simulink model "SVPWM_Simulation"  (R2018a)
settings: Solver=ode5  StartTime=0.0  StopTime=10  FixedStep=50e-6  MaxStep=1e-6  RelTol=1e-3  EnableMultiTasking=on
PostLoadFcn:
  | , if any(exist('dsrtsu_mdlpostloadfcn', 'file') == [2, 3, 6]), try dsrtsu_mdlpostloadfcn('Execute', bdroot); catch fprintf('Error in PostLoadFcn (dsrtsu_mdlpostloadfcn) for model "%s":\n %s\n', bdroot, lasterr); end, end,
InitFcn:
  | clear;
  | clc;
libraries: powerlib x8, simulink x1
settings Model: DSRTSU_INTERNAL_RTI_VER=510  DSRTSU_INTERNAL_RTI_TYPE=rti1104  RTICANMMDATA=struct('GeneralSetupData',struct('modelroot','C:\Users\elec\Desktop\SVPWM_1','generalsettings',struct('filesettings',struct('destfolder',struct('Name','RTICANMM_FILES','Check',1),'buildfolder',struct('Name','.','Check',1),'AbsDestfolder',struct('Name','C:\Users\elec\Desktop\SVPWM_1\RTICANMM_FILES'),'AbsBuildfolder',struct('Name','C:\Users\elec\Desktop\SVPWM_1'))),'options',struct('addpaths',1,'rmpaths',1,'addtrcexclusion',logical(1),'cannavigator',struct('checkmonitoring',0),'show_usrtrc',0,'use_usrtrc',0),'advanced',struct('options',[1 1 1 1 1 1 1 1 1 1 1 1 1 1 1 1 1 1 1 1 1 1 1 1 1 1 1 1 1 1 1 1 1 1 1 1 1 1 1 1 1 1 1 1 1 1 1 1 1 1 1 1 1 1 1 1 1 1 1 1 1 1 1 1 1 1 1 1 1 1 1 1 1 1 1 1 1 1 1 1 1 1 1 1 1 1 1 1 1 1 1 1 1 1 1 1 1 1 1 1]),'MPSetup',{{}},'modelname','shashank','block','shashank'))  DSRTSU_INTERNAL_RTIFLEXRAYCONFIG=110  DSRTSU_INTERNAL_RTIFPGA=110  Creator=HP  LastModifiedBy=asus
settings DataIOCC: LimitDataPoints=on  SaveFormat=Array
settings OptimizationCC: BlockReduction=off  ExpressionDepthLimit=2147483647
settings DebuggingCC: UnderspecifiedInitializationDetection=Classic  MergeDetectMultiDrivingBlocksExec=none  SolverPrmCheckMsg=warning  FcnCallInpInsideContextMsg=warning  StateNameClashWarn=warning  SFUnexpectedBacktrackingDiag=warning  SFNoUnconditionalDefaultTransitionDiag=warning  SFExecutionAtInitializationDiag=none
settings HardwareCC: ProdBitPerPointer=32  ProdBitPerSizeT=32  ProdBitPerPtrDiffT=32  ProdLargestAtomicInteger=Integer  ProdEndianess=BigEndian  ProdWordSize=32  ProdHWDeviceType=Custom Processor->Custom  TargetIntDivRoundTo=Zero  TargetEndianess=BigEndian  TargetHWDeviceType=Custom Processor->Custom
settings ModelReferenceCC: PropagateSignalLabelsOutOfModel=off
settings SFSimCC: MATLABDynamicMemAlloc=off
settings RTWCC: SystemTargetFile=rti1104.tlc  MakeCommand=make_rti  TemplateMakefile=rti1104.tmf  Description=dSPACE DS1104 Hardware Platform
settings CodeAppCC: StateflowObjectComments=on
settings STFCustomTargetCC: ParMdlRefBuildCompliant=on  GRTInterface=off  SystemTargetFile=rti1104.tlc
settings GRTTargetCC: TargetLangStandard=C89/C90 (ANSI)  CompOptLevelCompliant=off  ConcurrentExecutionCompliant=off  CombineOutputUpdateFcns=off  MatFileLogging=off  CPPClassGenCompliant=off  UseToolchainInfoCompliant=off
settings ConfigComp: CovMetricSettings=dw  CovHtmlReporting=on  CovSaveCumulativeToWorkspaceVar=on  CovSaveSingleToWorkspaceVar=on  CovExternalEMLEnable=off
settings SimscapeCC: SimscapeNormalizeSystem=off

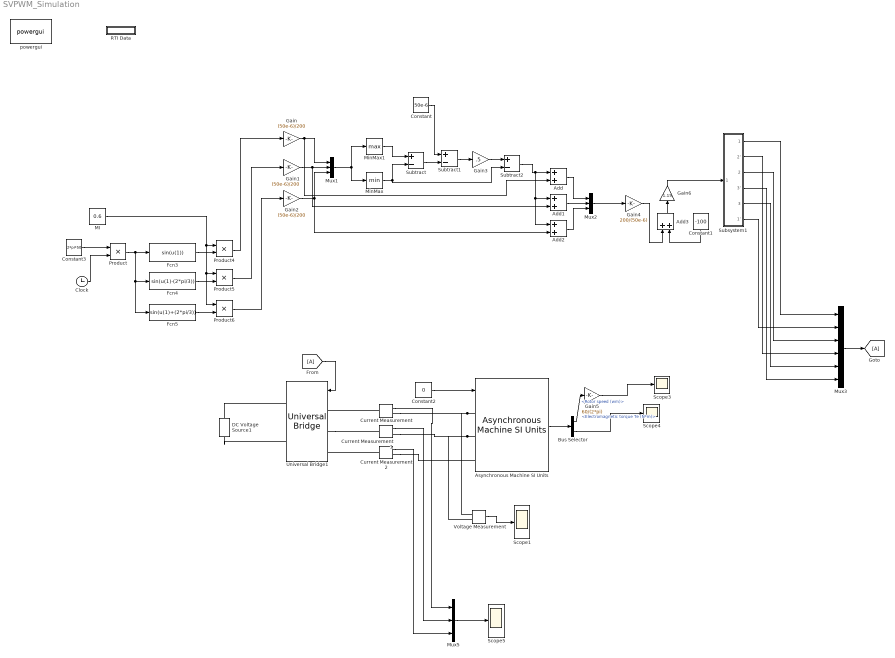
== system SVPWM_Simulation ==
  Add{,1..3} (4 alike) : Sum
  Asynchronous Machine SI Units : powerlib/Machines/Asynchronous Machine SI Units  RotorType=Squirrel-cage  PresetModel=No  MechanicalLoad=Torque Tm  ShowDetailedParameters=on  ReferenceFrame=Rotor  Units=SI  MeasurementBus=off  NominalParameters=[1300 415 50]  Stator=[14.15 0.0435]  Rotor=[4.36 0.0435]  Cage1=[ 0.022 0.226/377]  Cage2=[ 0.022 0.226/377]  Lm=0.59  Mechanical=[0.0131 0.002985 2]  PolePairs=2  InitialConditions=[1 0 0 0 0 0 0 0]  SimulateSaturation=off  Saturation=[14.03593122, 27.81365428, 53.79336849, 72.68890987, 97.98006896, 148.6815601, 215.7428561, 302.9841135, 428.7778367 ; 230, 322, 414, 460, 506, 552, 598, 644, 690]  LoadFlowParameters=1492000  TsPowergui=0  TsBlock=-1  IterativeModel=Trapezoidal non iterative  IterativeDiscreteModel=Trapezoidal non iterative  Pmec=0
  Bus Selector : BusSelector  OutputSignals=Mechanical.Rotor speed (wm),Mechanical.Electromagnetic torque Te (N*m)
  Clock : Clock
  Constant : Constant  Value=50e-6
  Constant1 : Constant  Value=-100
  Constant2 : Constant  Value=0
  Constant3 : Constant  Value=2*pi*50
  Current Measurement : powerlib/Measurements/Current Measurement  PhasorSimulation=off  OutputType=Complex  PSBequivalent=0
  Current Measurement1 : powerlib/Measurements/Current Measurement  PhasorSimulation=off  OutputType=Complex  PSBequivalent=0
  Current Measurement2 : powerlib/Measurements/Current Measurement  PhasorSimulation=off  OutputType=Complex  PSBequivalent=0
  DC Voltage Source1 : powerlib/Electrical Sources/DC Voltage Source  Amplitude=200  Measurements=None
  Fcn3 : Fcn  Expr=sin(u(1))
  Fcn4 : Fcn  Expr=sin(u(1)-(2*pi/3))
  Fcn5 : Fcn  Expr=sin(u(1)+(2*pi/3))
  Gain : Gain  Gain=(50e-6)/200
  Gain1 : Gain  Gain=(50e-6)/200
  Gain2 : Gain  Gain=(50e-6)/200
  Gain3 : Gain  Gain=.5
  Gain4 : Gain  Gain=200/(50e-6)
  Gain5 : Gain  Gain=60/(2*pi)
  Gain6 : Gain  Gain=1.15
  MI : Constant  Value=0.6
  MinMax : MinMax
  MinMax1 : MinMax  Function=max
  Mux1 : Mux  Inputs=3
  Mux2 : Mux  Inputs=3
  Mux3 : Mux  Inputs=6
  Mux5 : Mux  Inputs=3
  Product : Product
  Product4 : Product  RndMeth=Zero
  Product5 : Product  RndMeth=Zero
  Product6 : Product  RndMeth=Zero
  RTI Data : Subsystem  Tag=struct('RTIDataServer',struct('RTIDataServerVs','2','RTIModelDescription','struct(''main'',''shashank_load'',''sub'',''shashank_load'',''isMp'',0)'))  LoadFcn="if exist('rtidc'), try,  rtidc('DataHostBlockClbLoad', gcbh); catch, disp(['Warning: ''LoadFcn'' for RTI Data block failed: ' lasterr]); end, end,"  mask(RTI_DATA_HOST){}
      mask help:
      | RTI Data Block.
      | This block is used by RTI to store internal model-dependent data.
      | Please keep this block on the root level of the model. Deleting this block will result in data loss.
      |
      | NEVER DELETE OR COPY THIS BLOCK!
      settings: CopyFcn="if exist('rtidc'), try,  rtidc('DataHostBlockClbCopy', gcbh); catch, disp(['Warning: ''CopyFcn'' for RTI Data block failed: ' lasterr]); end, end,"  DeleteFcn="if exist('rtidc'), try,  rtidc('DataHostBlockClbDelete', gcbh); catch, disp(['Warning: ''DeleteFcn'' for RTI Data block failed: ' lasterr]); end, end,"  ModelCloseFcn="if exist('rtidc'), try,  rtidc('DataHostBlockClbModelClose', gcbh); catch, disp(['Warning: ''ModelCloseFcn'' for RTI Data block failed: ' lasterr]); end, end,"  PreSaveFcn="if exist('rtidc'), try,  rtidc('DataHostBlockClbPreSave', gcbh); catch, disp(['Warning: ''PreSaveFcn'' for RTI Data block failed: ' lasterr]); end, end,"  PostSaveFcn="if exist('rtidc'), try,  rtidc('DataHostBlockClbPostSave', gcbh); catch, disp(['Warning: ''PostSaveFcn'' for RTI Data block failed: ' lasterr]); end, end,"  NameChangeFcn="if exist('rtidc'), try,  rtidc('DataHostBlockClbNameChange', gcbh); catch, disp(['Warning: ''NameChangeFcn'' for RTI Data block failed: ' lasterr]); end, end,"
      mask Help:
      | RTI Data Block.
      | This block is used by RTI to store internal model-dependent data.
      | Please keep this block on the root level of the model. Deleting this block will result in data loss.
      | 
      | NEVER DELETE OR COPY THIS BLOCK!
      mask Display:
      | text(0.5, 0.5, 'RTI Data', 'HorizontalAlignment', 'center');
      | plot([1 0]);
  Scope{1,3..5} (4 alike) : Scope
  Subsystem1 : Subsystem
  Subtract : Sum  Inputs=+-
  Subtract1 : Sum  Inputs=+-
  Subtract2 : Sum  Inputs=+-
  Universal Bridge1 : powerlib/Power Electronics/Universal Bridge  Arms=3  SnubberResistance=1e5  SnubberCapacitance=inf  Device=IGBT / Diodes  Ron=1e-3  Lon=0  ForwardVoltages="[  0  0  ]"  ForwardVoltage=0  GTOparameters=[ 10e-6 , 20e-6 ]  IGBTparameters=[ 1e-6 , 2e-6 ]  Measurements=None  Measurements_2=None  converterType=Rectifier
  Voltage Measurement : powerlib/Measurements/Voltage Measurement  PhasorSimulation=off  OutputType=Complex  PSBequivalent=0
  powergui : powerlib/powergui  Priority=1  SimulationMode=Discrete  SampleTime=50e-6  frequency=60  Iterations=50  frequencyindice=0  Pbase=100e6  ErrMax=1e-4  UnitsV=kV  UnitsW=MW  buscounter=0  FunctionMessages=off  echomessages=off  EnableUseOfTLC=off  CurrentSourceSwitches=off  DisableSnubberDevices=off  DisableRonSwitches=off  DisableVfSwitches=off  DisplayEquations=off  SolverType=Tustin  Interpol=off  ExternalGateDelay=off  methode=off  Ts=0  x0status=blocks  SPID=off  SwTol=0  HookPort=off  RestoreLinks=warning  ResistiveCurrentMeasurement=off  Frange=[0:2:500]  Ylog=off  Xlog=on  ShowGrid=off  save=off  variable=ZData  structure=a5  ZoomFFT=off  StartTime=.2  cycles=3  DisplayStyle=2  fundamental=50  FreqAxis=on  MaxFrequency=1000  frequencyindicesteady=1  RmsSteady=1  display=off
  wires:
  Subtract1/1 -> Gain3/1
  Constant3/1 -> Product/1
  Mux1/1 -> MinMax1/1, MinMax/1
  MI/1 -> Product6/1, Product5/1, Product4/1
  Fcn5/1 -> Product6/2
  Product/1 -> Fcn5/1, Fcn4/1, Fcn3/1
  MinMax/1 -> Subtract/2, Subtract2/2
  Fcn4/1 -> Product5/2
  Product4/1 -> Gain/1
  Gain1/1 -> Mux1/2, Add1/2
  Constant1/1 -> Add3/2
  Clock/1 -> Product/2
  Gain2/1 -> Mux1/3, Add2/2
  Mux2/1 -> Gain4/1
  Subtract2/1 -> Add/1, Add1/1, Add2/1
  MinMax1/1 -> Subtract/1
  Gain6/1 -> Subsystem1/1(In1)
  Gain4/1 -> Add3/1
  Gain/1 -> Mux1/1, Add/2
  Fcn3/1 -> Product4/2
  Add/1 -> Mux2/1
  Add1/1 -> Mux2/2
  Add3/1 -> Gain6/1
  Constant/1 -> Subtract1/1
  Add2/1 -> Mux2/3
  Gain3/1 -> Subtract2/1
  Product5/1 -> Gain1/1
  Subtract/1 -> Subtract1/2
  Product6/1 -> Gain2/1
  Subsystem1/1(1) -> Mux3/1
  Subsystem1/6(1') -> Mux3/2
  Subsystem1/3(2) -> Mux3/3
  Subsystem1/2(2') -> Mux3/4
  Subsystem1/5(3) -> Mux3/5
  Subsystem1/4(3') -> Mux3/6
  Bus Selector/2 -> Scope4/1  "<Electromagnetic torque Te (N*m)>"
  [A] -> Universal Bridge1/1
  Voltage Measurement/1 -> Scope1/1
  Bus Selector/1 -> Gain5/1  "<Rotor speed (wm)>"
  Constant2/1 -> Asynchronous Machine SI Units/1
  Current Measurement2/1 -> Mux5/3
  Asynchronous Machine SI Units/1 -> Bus Selector/1
  Mux5/1 -> Scope5/1
  Current Measurement1/1 -> Mux5/2
  Gain5/1 -> Scope3/1
  Current Measurement/1 -> Mux5/1
  Mux3/1 -> [A]
  connections:
  Asynchronous Machine SI Units/LConn2 -- Current Measurement1/RConn1 -- Voltage Measurement/LConn2
  Asynchronous Machine SI Units/LConn1 -- Current Measurement/RConn1 -- Voltage Measurement/LConn1
  DC Voltage Source1/RConn1 -- Universal Bridge1/RConn1
  DC Voltage Source1/LConn1 -- Universal Bridge1/RConn2
  Current Measurement2/RConn1 -- Asynchronous Machine SI Units/LConn3
  Current Measurement/LConn1 -- Universal Bridge1/LConn1
  Universal Bridge1/LConn2 -- Current Measurement1/LConn1
  Current Measurement2/LConn1 -- Universal Bridge1/LConn3

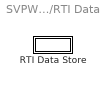
== system SVPWM_Simulation/RTI Data ==
  RTI Data Store : Subsystem  Tag="struct('private',struct('version',struct('dsVer',uint32(2),'dsVerCreation',uint32(2),'RTI',struct('ver','7.9','type','RTI1104')),'access',struct('type','Model','isPerm',1,'created',['06-Dec-2017 13:33:18'],'modified',['06-Nov-2017 16:43:46'],'location','')),'public',struct('main',struct('data',[]),'sub',struct('name',{{'shashank_load'}},'data',{{struct('TH',struct('thTaskInfo',struct('taskType',{'TIMER','HWINT','TMRINT','SWINT','GLINT'},'tasksNumOf',{1,0,0,0,0},'srcIds',{{'TIMERA'},{},{},{},{}},'taskNames',{{['Timer Task 1']},{},{},{},{}})),'th_tc',struct('dataType','TASK','taskGroupId','','taskGroupList',{{}},'taskSchedulingPolicy','FCFS','taskType','TIMER','blkh',-1,'srcId','TIMERA','srcSgnName',['Timer A interrupt'],'srcCpuName','','taskName',['Timer Task 1  [5e-05] s'],'taskNameDisplayExt','','smplTime',5e-5,'smplTimeOffs',0,'hasFixedPriority',0,'priority',1,'hasFixedOvc',0,'ovcType',1,'ovcMax',1),'tc_th',struct('dataType','TASK','taskGroupId','','taskGroupList',{{}},'taskSchedulingPolicy','FCFS','taskType','TIMER','blkh',-1,'srcId','TIMERA','srcSgnName',['Timer A interrupt'],'srcCpuName','','taskName',['Timer Task 1  [5e-05] s'],'taskNameDisplayExt','','smplTime',5e-5,'smplTimeOffs',0,'hasFixedPriority',0,'priority',1,'hasFixedOvc',0,'ovcType',1,'ovcMax',1))}})))"  mask(RTI_DATA_STORE){}
      mask help:
      | RTI Data Store Block. This block is used by RTI to store internal model dependent data. Deleting this block will result in data loss.
      |
      | NEVER DELETE, COPY, OR MODIFY THIS BLOCK!
      mask Help:
      | RTI Data Store Block. This block is used by RTI to store internal model dependent data. Deleting this block will result in data loss.
      | 
      | NEVER DELETE, COPY, OR MODIFY THIS BLOCK!
      mask Display: text(0.5, 0.5, ' ', 'HorizontalAlignment', 'center');

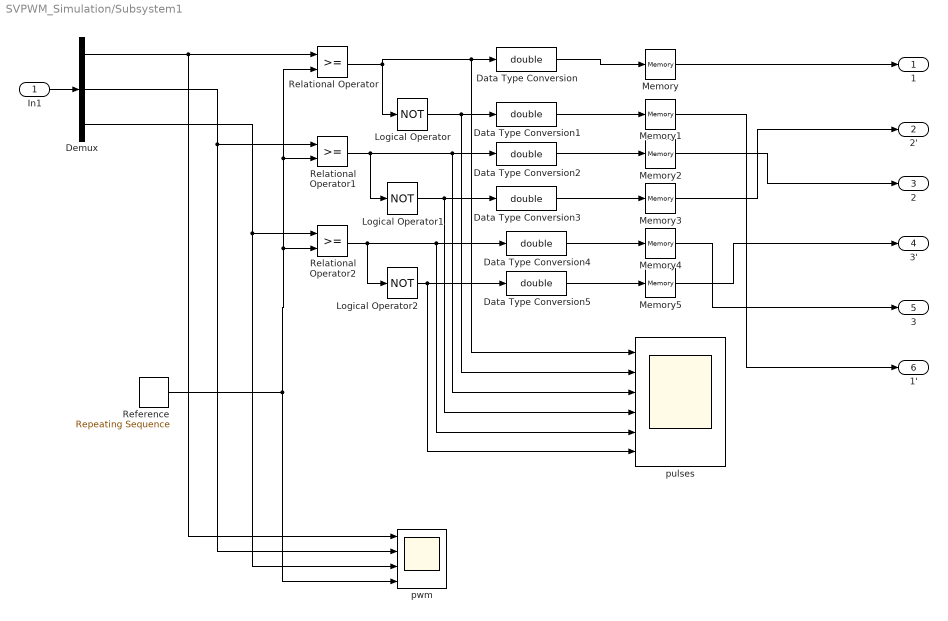
== system SVPWM_Simulation/Subsystem1 ==
  In1 : Inport
  Data Type Conversion{,1..5} (6 alike) : DataTypeConversion  OutDataTypeStr=double
  Demux : Demux  Outputs=3
  Logical Operator : Logic  Operator=NOT  AllPortsSameDT=off  OutDataTypeStr=boolean
  Logical Operator1 : Logic  Operator=NOT  AllPortsSameDT=off  OutDataTypeStr=boolean
  Logical Operator2 : Logic  Operator=NOT  AllPortsSameDT=off  OutDataTypeStr=boolean
  Memory{,1..5} (6 alike) : Memory
  Reference : simulink/Sources/Repeating Sequence  rep_seq_t=[0 1/2000 1/1000]  rep_seq_y=[-1 1 -1]
  Relational Operator : RelationalOperator  OutDataTypeStr=boolean  RndMeth=Nearest
  Relational Operator1 : RelationalOperator  OutDataTypeStr=boolean  RndMeth=Nearest
  Relational Operator2 : RelationalOperator  OutDataTypeStr=boolean  RndMeth=Nearest
  pulses : Scope  NumInputPorts=6
  pwm : Scope  NumInputPorts=4
  1 : Outport
  2' : Outport  Port=2
  2 : Outport  Port=3
  3' : Outport  Port=4
  3 : Outport  Port=5
  1' : Outport  Port=6
  wires:
  Memory4/1 -> 3/1
  Memory1/1 -> 1'/1
  Memory3/1 -> 2'/1
  Memory/1 -> 1/1
  Memory2/1 -> 2/1
  In1/1 -> Demux/1
  Memory5/1 -> 3'/1
  Data Type Conversion4/1 -> Memory4/1
  Demux/1 -> pwm/1, Relational Operator/1
  Data Type Conversion1/1 -> Memory1/1
  Reference/1 -> pwm/4, Relational Operator/2, Relational Operator1/2, Relational Operator2/2
  Demux/3 -> pwm/3, Relational Operator2/1
  Data Type Conversion2/1 -> Memory2/1
  Data Type Conversion/1 -> Memory/1
  Relational Operator1/1 -> pulses/3, Data Type Conversion2/1, Logical Operator1/1
  Logical Operator1/1 -> pulses/4, Data Type Conversion3/1
  Logical Operator2/1 -> pulses/6, Data Type Conversion5/1
  Relational Operator/1 -> pulses/1, Data Type Conversion/1, Logical Operator/1
  Demux/2 -> pwm/2, Relational Operator1/1
  Relational Operator2/1 -> pulses/5, Data Type Conversion4/1, Logical Operator2/1
  Logical Operator/1 -> pulses/2, Data Type Conversion1/1
  Data Type Conversion5/1 -> Memory5/1
  Data Type Conversion3/1 -> Memory3/1

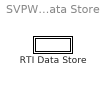
== system SVPWM_Simulation/RTI Data/RTI Data Store ==
  RTI Data Store : Subsystem  mask(RTI_DATA_STORE){}
      mask help:
      | RTI Data Store Block. This block is used by RTI to store internal model dependent data. Deleting this block will result in data loss.
      |
      | NEVER DELETE, COPY, OR MODIFY THIS BLOCK!
      mask Help:
      | RTI Data Store Block. This block is used by RTI to store internal model dependent data. Deleting this block will result in data loss.
      | 
      | NEVER DELETE, COPY, OR MODIFY THIS BLOCK!
      mask Display: text(0.5, 0.5, ' ', 'HorizontalAlignment', 'center');

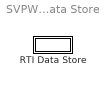
== system SVPWM_Simulation/RTI Data/RTI Data Store/RTI Data Store ==
  RTI Data Store : Subsystem  mask(RTI_DATA_STORE){}
      mask help:
      | RTI Data Store Block. This block is used by RTI to store internal model dependent data. Deleting this block will result in data loss.
      |
      | NEVER DELETE, COPY, OR MODIFY THIS BLOCK!
      mask Help:
      | RTI Data Store Block. This block is used by RTI to store internal model dependent data. Deleting this block will result in data loss.
      | 
      | NEVER DELETE, COPY, OR MODIFY THIS BLOCK!
      mask Display: text(0.5, 0.5, ' ', 'HorizontalAlignment', 'center');

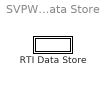
== system SVPWM_Simulation/RTI Data/RTI Data Store/RTI Data Store/RTI Data Store ==
  RTI Data Store : Subsystem  mask(RTI_DATA_STORE){}
      mask help:
      | RTI Data Store Block. This block is used by RTI to store internal model dependent data. Deleting this block will result in data loss.
      |
      | NEVER DELETE, COPY, OR MODIFY THIS BLOCK!
      mask Help:
      | RTI Data Store Block. This block is used by RTI to store internal model dependent data. Deleting this block will result in data loss.
      | 
      | NEVER DELETE, COPY, OR MODIFY THIS BLOCK!
      mask Display: text(0.5, 0.5, ' ', 'HorizontalAlignment', 'center');

== system SVPWM_Simulation/RTI Data/RTI Data Store/RTI Data Store/RTI Data Store/RTI Data Store ==
